simulink model "ricontinuousmode0x5B20x5D"  (R2025a)
settings: Solver=VariableStepAuto  StartTime=0.0  StopTime=2  FixedStep=5e-6  RelTol=1e-3
libraries: spsIdealSwitchLib x12, spsSeriesRLCBranchLib x5, spsGroundLib x2, spsVoltageMeasurementLib x2, spsDCVoltageSourceLib x1, sps_lib x1
settings Model: Creator=baish  LastModifiedBy=91969
settings RTWCC: GPUComputeCapability=3.5

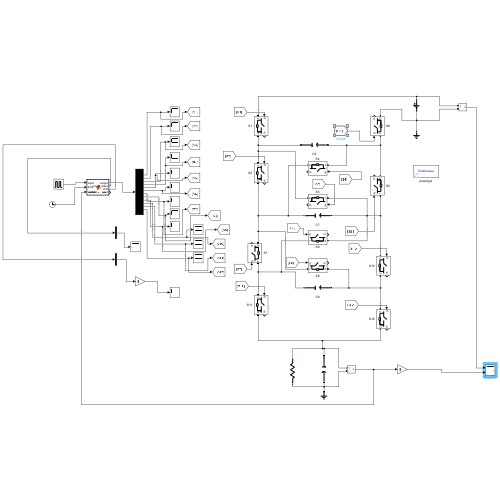
[thumbnail: Simulink's stored preview of the top-level diagram]
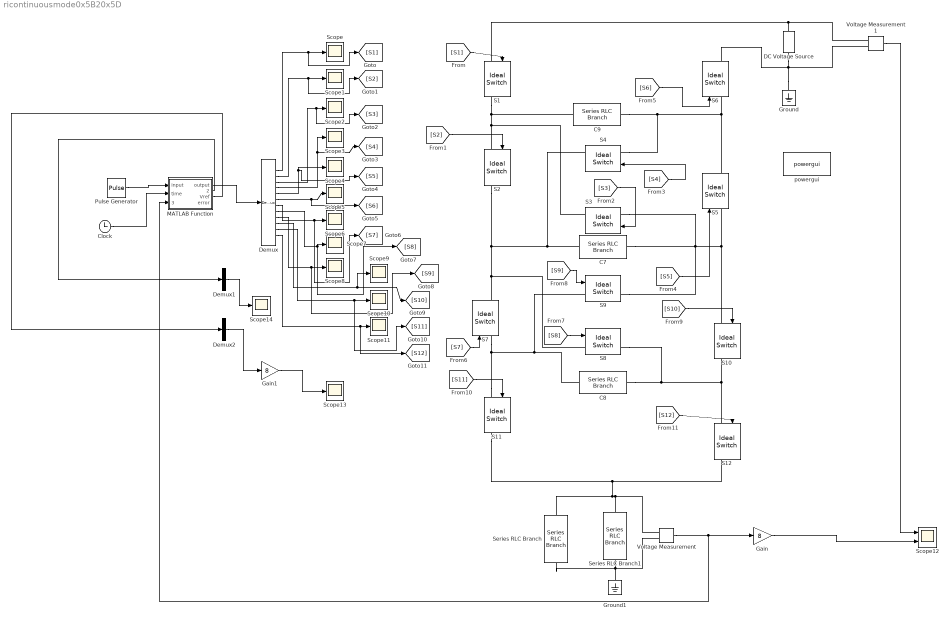
== system ricontinuousmode0x5B20x5D ==
  C7 : spsSeriesRLCBranchLib/Series RLC Branch  LConnTagsString=__new0  RConnTagsString=__new0  BranchType=C  Resistance=1  Inductance=1e-3  SetiL0=off  InitialCurrent=0  Capacitance=10e-6  Setx0=off  InitialVoltage=0  Measurements=None
  C8 : spsSeriesRLCBranchLib/Series RLC Branch  LConnTagsString=__new0  RConnTagsString=__new0  BranchType=C  Resistance=1  Inductance=1e-3  SetiL0=off  InitialCurrent=0  Capacitance=10e-6  Setx0=off  InitialVoltage=0  Measurements=None
  C9 : spsSeriesRLCBranchLib/Series RLC Branch  LConnTagsString=__new0  RConnTagsString=__new0  BranchType=C  Resistance=1  Inductance=1e-3  SetiL0=off  InitialCurrent=0  Capacitance=10e-6  Setx0=off  InitialVoltage=0  Measurements=None
  Clock : Clock
  DC Voltage Source : spsDCVoltageSourceLib/DC Voltage Source  Amplitude=8  Measurements=None
  Demux : Demux  Outputs=12
  Demux1 : Demux  Outputs=1
  Demux2 : Demux  Outputs=1
  Gain : Gain  Gain=8
  Gain1 : Gain  Gain=8
  Ground : spsGroundLib/Ground  LConnTagsString=a
  Ground1 : spsGroundLib/Ground  LConnTagsString=a
  MATLAB Function : MATLAB Function  TreatAsAtomicUnit=on
  Pulse Generator : DiscretePulseGenerator  PulseType=Time based  Period=1/(10e3)  PulseWidth=50
  S{1..12} (12 alike) : spsIdealSwitchLib/Ideal Switch  Ron=0.001  Lon=0  IC=0  Rs=1e5  Cs=inf  Measurements=on
  Scope{,1..11,13..14} (14 alike) : Scope
      Scope settings: TimeSpan=0.0002  TimeDisplayOffset=2.632  ActiveDisplayYMinimum=-0.125  ActiveDisplayYMaximum=1.125
      Scope1 settings: TimeSpan=0.0002  TimeDisplayOffset=2.632  ActiveDisplayYMinimum=-0.125  ActiveDisplayYMaximum=1.125  DataLoggingVariableName=ScopeData2
      Scope10 settings: TimeSpan=0.0002  TimeDisplayOffset=2.632  ActiveDisplayYMinimum=-0.125  ActiveDisplayYMaximum=1.125  DataLoggingVariableName=ScopeData3
      Scope11 settings: TimeSpan=0.0002  TimeDisplayOffset=2.632  ActiveDisplayYMinimum=-0.125  ActiveDisplayYMaximum=1.125  DataLoggingVariableName=ScopeData4
      Scope13 settings: ActiveDisplayYMinimum=-0.78643  ActiveDisplayYMaximum=7.86219
      Scope14 settings: ActiveDisplayYMinimum=-1  ActiveDisplayYMaximum=19  DataLoggingVariableName=ScopeData2
      Scope2 settings: TimeSpan=0.0002  TimeDisplayOffset=2.632  ActiveDisplayYMinimum=-0.125  ActiveDisplayYMaximum=1.125  DataLoggingVariableName=ScopeData6
      Scope3 settings: TimeSpan=0.0002  TimeDisplayOffset=2.632  ActiveDisplayYMinimum=-0.125  ActiveDisplayYMaximum=1.125  DataLoggingVariableName=ScopeData7
      Scope4 settings: TimeSpan=0.0002  TimeDisplayOffset=2.632  ActiveDisplayYMinimum=-0.125  ActiveDisplayYMaximum=1.125  DataLoggingVariableName=ScopeData8
      Scope5 settings: TimeSpan=0.0002  TimeDisplayOffset=2.632  ActiveDisplayYMinimum=-0.125  ActiveDisplayYMaximum=1.125  DataLoggingVariableName=ScopeData9
      Scope6 settings: TimeSpan=0.0002  TimeDisplayOffset=2.632  ActiveDisplayYMinimum=-0.125  ActiveDisplayYMaximum=1.125  DataLoggingVariableName=ScopeData10
      Scope7 settings: TimeSpan=0.0002  TimeDisplayOffset=2.632  ActiveDisplayYMinimum=-0.125  ActiveDisplayYMaximum=1.125  DataLoggingVariableName=ScopeData11
      Scope8 settings: TimeSpan=0.0002  TimeDisplayOffset=2.632  ActiveDisplayYMinimum=-0.125  ActiveDisplayYMaximum=1.125  DataLoggingVariableName=ScopeData12
      Scope9 settings: TimeSpan=0.0002  TimeDisplayOffset=2.632  ActiveDisplayYMinimum=-0.125  ActiveDisplayYMaximum=1.125
  Scope12 : Scope  NumInputPorts=2
      settings: ActiveDisplayYMinimum=-0.76994  ActiveDisplayYMaximum=8.97444  DataLoggingVariableName=ScopeData5
  Series RLC Branch : spsSeriesRLCBranchLib/Series RLC Branch  LConnTagsString=__new0  RConnTagsString=__new0  BranchType=R  Resistance=3000  Inductance=1e-3  SetiL0=off  InitialCurrent=0  Capacitance=1e-6  Setx0=off  InitialVoltage=0  Measurements=None
  Series RLC Branch1 : spsSeriesRLCBranchLib/Series RLC Branch  LConnTagsString=__new0  RConnTagsString=__new0  BranchType=C  Resistance=1  Inductance=1e-3  SetiL0=off  InitialCurrent=0  Capacitance=1000e-6  Setx0=off  InitialVoltage=0  Measurements=None
  Voltage Measurement : spsVoltageMeasurementLib/Voltage Measurement  PhasorSimulation=off  OutputType=Complex  PSBequivalent=0
  Voltage Measurement1 : spsVoltageMeasurementLib/Voltage Measurement  PhasorSimulation=off  OutputType=Complex  PSBequivalent=0
  powergui : sps_lib/powergui  Priority=1  SimulationMode=Continuous  SampleTime=5e-6  frequency=60  Iterations=50  frequencyindice=0  Pbase=100e6  ErrMax=1e-4  UnitsV=kV  UnitsW=MW  buscounter=0  FunctionMessages=off  echomessages=off  EnableUseOfTLC=off  CurrentSourceSwitches=off  DisableSnubberDevices=off  DisableRonSwitches=off  DisableVfSwitches=off  DisplayEquations=off  AutomaticDiscreteSolvers=off  SolverType=Tustin/Backward Euler (TBE)  Interpol=off  ExternalGateDelay=off  methode=off  Ts=100  x0status=blocks  SPID=on  SwTol=0  HookPort=off  NonlinearTolerance=1e-4  nMaxIteration=100  ContinueOnMaxIteration=off  RestoreLinks=warning  ResistiveCurrentMeasurement=off  Frange=[0:2:500]  Ylog=off  Xlog=on  ShowGrid=off  save=off  variable=ZData  structure=0  ZoomFFT=off  StartTime=0.0  cycles=1  DisplayStyle=1  fundamental=60  FreqAxis=off  MaxFrequency=1000  frequencyindicesteady=1  RmsSteady=1  display=off
  wires:
  Demux/2 -> [S2], Scope1/1
  Demux/1 -> [S1], Scope/1
  Demux/3 -> [S3], Scope2/1
  Demux/8 -> [S8], Scope7/1
  MATLAB Function/1(output) -> Demux/1
  [S12] -> S12/1
  Demux/9 -> [S9], Scope8/1
  [S11] -> S11/1
  Demux/11 -> [S11], Scope10/1
  [S5] -> S5/1
  [S1] -> S1/1
  Demux/4 -> Scope3/1, [S4]
  [S4] -> S4/1
  Demux/12 -> [S12], Scope11/1
  Demux/7 -> [S7], Scope6/1
  [S3] -> S3/1
  [S8] -> S8/1
  [S10] -> S10/1
  Demux/5 -> [S5], Scope4/1
  Pulse Generator/1 -> MATLAB Function/1(input)
  [S7] -> S7/1
  [S6] -> S6/1
  [S2] -> S2/1
  [S9] -> S9/1
  Demux/10 -> Scope9/1, [S10]
  Voltage Measurement/1 -> Gain/1, MATLAB Function/3(Vactual)
  Demux/6 -> [S6], Scope5/1
  Clock/1 -> MATLAB Function/2(time)
  Gain/1 -> Scope12/2
  Demux1/1 -> Scope14/1
  Demux2/1 -> Gain1/1
  Gain1/1 -> Scope13/1
  MATLAB Function/2(mode_index) -> Demux1/1
  MATLAB Function/3(Vref) -> Demux2/1
  Voltage Measurement1/1 -> Scope12/1
  connections:
  S5/LConn1 -- S10/LConn1 -- S9/RConn1 -- S3/LConn1 -- C7/RConn1
  C9/LConn1 -- S1/RConn1 -- S3/RConn1 -- S2/LConn1
  C7/LConn1 -- S4/RConn1 -- S2/RConn1 -- S8/LConn1 -- S7/RConn1
  Voltage Measurement/LConn1 -- S11/RConn1 -- S12/RConn1 -- Series RLC Branch/LConn1 -- Series RLC Branch1/LConn1
  C8/RConn1 -- S8/RConn1 -- S12/LConn1 -- S10/RConn1
  Ground/LConn1 -- Voltage Measurement1/LConn2 -- DC Voltage Source/LConn1 -- S6/RConn1
  S11/LConn1 -- S7/LConn1 -- S9/LConn1 -- C8/LConn1
  S6/LConn1 -- S5/RConn1 -- S4/LConn1 -- C9/RConn1
  Ground1/LConn1 -- Series RLC Branch/RConn1 -- Voltage Measurement/LConn2 -- Series RLC Branch1/RConn1
  S1/LConn1 -- Voltage Measurement1/LConn1 -- DC Voltage Source/RConn1

== matlab function ricontinuousmode0x5B20x5D/MATLAB Function ==
  settings: updateMethod=DISCRETE  sampleTime=5e-6
  data: input input; output output double size=12; time input; Vactual input; mode_index output; Vref output; error output
function [output, mode_index, Vref, error] = switch_control(input, time, Vactual)
    persistent a cnt integral_error prev_error mode_select_persist
    if isempty(a)
        a = zeros(12,1);
        cnt = 0;
        mode_select_persist = 1;
        integral_error = 0;
        prev_error = 0;
    end

    %–– Define all 17 switching patterns ––
    % 1/2
    SW38_half_1         = [0,1,0,0,0,1,1,0,0,0,1,0];
    SW38_half_2         = [1,0,0,0,1,0,0,0,0,1,0,1];
    % 1/3
    SW38_third_1        = [0,0,0,0,1,1,1,0,0,0,1,0];
    SW38_third_2        = [0,1,0,0,0,1,0,0,0,1,0,1];
    SW38_third_3        = [1,0,0,0,1,0,0,0,0,1,0,1];
    % 2/3
    SW38_two_third_1    = [0,1,0,0,0,1,1,0,0,0,1,0];
    SW38_two_third_2    = [1,0,0,0,1,0,1,0,0,0,1,0];
    SW38_two_third_3    = [1,1,0,0,0,0,0,0,0,1,0,1];
    % 1/5
    SW38_one_fifth_1    = [0,0,0,0,1,1,0,0,0,1,1,0];
    SW38_one_fifth_2    = [0,0,0,0,1,1,1,0,0,0,0,1];
    SW38_one_fifth_3    = [0,1,0,0,0,1,0,0,0,1,0,1];
    SW38_one_fifth_4    = [1,0,0,1,0,0,0,0,0,1,1,0];
    SW38_one_fifth_5    = [1,0,0,0,1,0,0,0,1,0,0,1];
    % 2/5
    SW38_two_fifth_1    = [0,0,0,0,1,1,1,0,0,0,1,0];
    SW38_two_fifth_2    = [0,1,0,0,0,1,0,0,0,1,1,0];
    SW38_two_fifth_3    = [0,1,0,0,0,1,1,0,0,0,0,1];
    SW38_two_fifth_4    = [1,0,0,0,1,0,0,0,0,1,0,1];
    % 4/5
    SW38_four_fifth_1   = [0,0,1,0,0,1,0,0,0,1,1,0];
    SW38_four_fifth_2   = [0,0,1,0,0,1,1,0,0,0,0,1];
    SW38_four_fifth_3   = [1,0,0,0,1,0,1,0,0,0,1,0];
    SW38_four_fifth_4   = [1,1,0,0,0,0,0,0,0,1,1,0];
    % 1/4
    SW38_one_fourth_1   = [0,0,0,0,1,1,1,0,0,0,1,0];
    SW38_one_fourth_2   = [0,1,0,0,0,1,0,0,0,1,0,1];
    SW38_one_fourth_3   = [1,0,0,1,0,0,0,0,0,1,0,1];
    % 3/4
    SW38_three_fourth_1 = [0,0,1,0,0,1,1,0,0,0,1,0];
    SW38_three_fourth_2 = [1,1,0,0,0,0,0,0,0,1,0,1];
    SW38_three_fourth_3 = [1,0,0,0,1,0,1,0,0,0,1,0];
    % 1/8
    SW38_one_eighth_1   = [0,0,0,0,1,1,0,0,0,1,1,0];
    SW38_one_eighth_2   = [0,0,0,0,1,1,1,0,0,0,0,1];
    SW38_one_eighth_3   = [0,1,0,0,0,1,0,0,1,0,0,1];
    SW38_one_eighth_4   = [1,0,0,1,0,0,0,0,1,0,0,1];
    % 3/8
    SW38_three_eighth_1 = [0,0,0,0,1,1,0,1,0,0,1,0];
    SW38_three_eighth_2 = [0,1,0,0,0,1,0,0,0,1,1,0];
    SW38_three_eighth_3 = [0,1,0,0,0,1,1,0,0,0,0,1];
    SW38_three_eighth_4 = [1,0,0,1,0,0,0,0,0,1,1,0];
    SW38_three_eighth_5 = [1,0,0,0,1,0,0,0,1,0,0,1];
    % 5/8
    SW38_five_eighth_1  = [0,1,0,0,0,1,0,1,0,0,1,0];
    SW38_five_eighth_2  = [0,0,1,0,0,1,1,0,0,0,0,1];
    SW38_five_eighth_3  = [1,1,0,0,0,0,0,0,1,0,0,1];
    SW38_five_eighth_4  = [1,0,0,0,1,0,0,0,0,1,1,0];
    SW38_five_eighth_5  = [1,0,0,0,1,0,1,0,0,0,0,1];
    % 7/8
    SW38_seven_eighth_1 = [0,0,1,0,0,1,0,1,0,0,1,0];
    SW38_seven_eighth_2 = [1,0,0,0,1,0,0,1,0,0,1,0];
    SW38_seven_eighth_3 = [1,1,0,0,0,0,0,0,0,1,1,0];
    SW38_seven_eighth_4 = [1,1,0,0,0,0,1,0,0,0,0,1];
    % 1/7
    SW38_one_seventh_1  = [0,0,0,0,1,1,0,0,0,1,1,0];
    SW38_one_seventh_2  = [0,0,0,0,1,1,1,0,0,0,0,1];
    SW38_one_seventh_3  = [0,1,0,0,0,1,0,0,1,0,0,1];
    SW38_one_seventh_4  = [1,0,0,1,0,0,0,0,0,1,0,1];
    % 3/7
    SW38_three_seventh_1 = [0,0,0,0,1,1,0,1,0,0,1,0];
    SW38_three_seventh_2 = [0,1,0,0,0,1,1,0,0,0,0,1];
    SW38_three_seventh_3 = [1,0,0,0,1,0,0,0,0,1,0,1];
    SW38_three_seventh_4 = [0,1,0,0,0,1,0,0,0,1,1,0];
    % 4/7
    SW38_four_seventh_1 = [0,1,0,0,0,1,1,0,0,0,1,0];
    SW38_four_seventh_2 = [1,0,0,0,1,0,0,0,0,1,1,0];
    SW38_four_seventh_3 = [1,0,0,0,1,0,1,0,0,0,0,1];
    SW38_four_seventh_4 = [1,1,0,0,0,0,0,0,1,0,0,1];
    % 5/7
    SW38_five_seventh_1 = [0,1,0,0,0,1,0,1,0,0,1,0];
    SW38_five_seventh_2 = [0,0,1,0,0,1,1,0,0,0,0,1];
    SW38_five_seventh_3 = [1,1,0,0,0,0,0,0,0,1,0,1];
    SW38_five_seventh_4 = [1,0,0,0,1,0,1,0,0,0,1,0];
    % 6/7
    SW38_six_seventh_1  = [0,0,1,0,0,1,1,0,0,0,1,0];
    SW38_six_seventh_2  = [1,1,0,0,0,0,0,0,0,1,1,0];
    SW38_six_seventh_3  = [1,1,0,0,0,0,1,0,0,0,0,1];
    SW38_six_seventh_4  = [1,0,0,0,1,0,0,1,0,0,1,0];

    %–– mode selection and PID feedback ––
    mode_index = mod(floor(time/10),17) + 1;
    mode_select_persist = mode_index;
    fractions = [1/2,1/3,2/3,1/5,2/5,4/5,1/4,3/4,1/8,3/8,5/8,7/8,1/7,3/7,4/7,5/7,6/7];
    Vref  = fractions(mode_index);
    error = Vref - Vactual;
    integral_error = integral_error + error;
    derivative = error - prev_error;
    Kp = 2.0; Ki = 10.0; Kd = 0.1;
    correction = Kp*error + Ki*integral_error + Kd*derivative;
    prev_error = error;
    if abs(correction) > 0.05
        cnt = 0;
    end

    %–– select pattern based on mode_index and cnt ––
    cnt = cnt + 1;
    switch mode_index
      case 1;  a = SW38_half_1;         if cnt>5,  a=SW38_half_2;           end
      case 2;  a = SW38_third_1;        if cnt>3,  a=SW38_third_2;        end; if cnt>6, a=SW38_third_3;  end
      case 3;  a = SW38_two_third_1;    if cnt>3,  a=SW38_two_third_2;    end; if cnt>6, a=SW38_two_third_3; end
      case 4;  a = SW38_one_fifth_1;     if cnt>2,  a=SW38_one_fifth_2;     end; if cnt>4, a=SW38_one_fifth_3; end; if cnt>6, a=SW38_one_fifth_4; end; if cnt>8, a=SW38_one_fifth_5; end
      case 5;  a = SW38_two_fifth_1;     if cnt>2,  a=SW38_two_fifth_2;     end; if cnt>4, a=SW38_two_fifth_3; end; if cnt>6, a=SW38_two_fifth_4; end
      case 6;  a = SW38_four_fifth_1;    if cnt>2,  a=SW38_four_fifth_2;    end; if cnt>4, a=SW38_four_fifth_3; end; if cnt>6, a=SW38_four_fifth_4; end
      case 7;  a = SW38_one_fourth_1;    if cnt>3,  a=SW38_one_fourth_2;    end; if cnt>6, a=SW38_one_fourth_3; end
      case 8;  a = SW38_three_fourth_1;  if cnt>3,  a=SW38_three_fourth_2;  end; if cnt>6, a=SW38_three_fourth_3; end
      case 9;  a = SW38_one_eighth_1;    if cnt>2,  a=SW38_one_eighth_2;    end; if cnt>4, a=SW38_one_eighth_3; end; if cnt>6, a=SW38_one_eighth_4; end
      case 10; a = SW38_three_eighth_1;  if cnt>2,  a=SW38_three_eighth_2;  end; if cnt>4, a=SW38_three_eighth_3; end; if cnt>6, a=SW38_three_eighth_4; end; if cnt>8, a=SW38_three_eighth_5; end
      case 11; a = SW38_five_eighth_1;   if cnt>2,  a=SW38_five_eighth_2;   end; if cnt>4, a=SW38_five_eighth_3; end; if cnt>6, a=SW38_five_eighth_4; end; if cnt>8, a=SW38_five_eighth_5; end
      case 12; a = SW38_seven_eighth_1;  if cnt>2,  a=SW38_seven_eighth_2;  end; if cnt>4, a=SW38_seven_eighth_3; end; if cnt>6, a=SW38_seven_eighth_4; end
      case 13; a = SW38_one_seventh_1;   if cnt>2,  a=SW38_one_seventh_2;   end; if cnt>4, a=SW38_one_seventh_3; end; if cnt>6, a=SW38_one_seventh_4; end
      case 14; a = SW38_three_seventh_1; if cnt>2,  a=SW38_three_seventh_2; end; if cnt>4, a=SW38_three_seventh_3; end; if cnt>6, a=SW38_three_seventh_4; end
      case 15; a = SW38_four_seventh_1;  if cnt>2,  a=SW38_four_seventh_2;  end; if cnt>4, a=SW38_four_seventh_3; end; if cnt>6, a=SW38_four_seventh_4; end
      case 16; a = SW38_five_seventh_1;  if cnt>2,  a=SW38_five_seventh_2;  end; if cnt>4, a=SW38_five_seventh_3; end; if cnt>6, a=SW38_five_seventh_4; end
      case 17; a = SW38_six_seventh_1;   if cnt>2,  a=SW38_six_seventh_2;   end; if cnt>4, a=SW38_six_seventh_3; end; if cnt>6, a=SW38_six_seventh_4; end
    end

    if cnt >= 10
        cnt = 0;
    end

    output = reshape(a, 12, 1);
end
